simulink model "subsysChanged"  (R2023b)
settings: Solver=VariableStepAuto  StartTime=0.0  StopTime=10.0  RelTol=1e-3
settings Model: Creator=neham  LastModifiedBy=neham

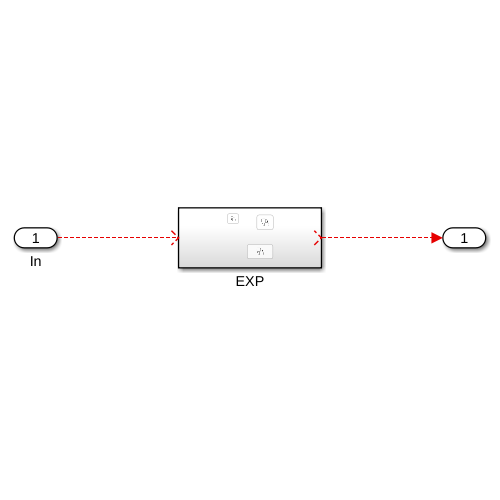
[thumbnail: Simulink's stored preview of the top-level diagram]
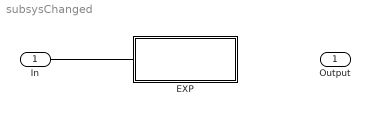
== system subsysChanged ==
  In : Inport
  EXP : Subsystem
  Output : Outport
  wires:
  ? -> Output/1
  In/1 -> ?

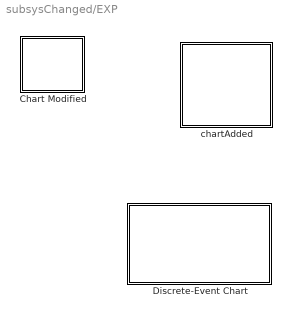
== system subsysChanged/EXP ==
  Chart Modified : Stateflow chart  TreatAsAtomicUnit=on
  Discrete-Event Chart : Stateflow chart  TreatAsAtomicUnit=on
  chartAdded : Stateflow chart  TreatAsAtomicUnit=on

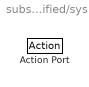
== system subsysChanged/EXP/Chart Modified/sys ==
  Action Port : ActionPort
      settings: CopyFcn=Stateflow.SLINSF.SimulinkMan.removeBlockPreDeleteFcn  PreDeleteFcn=Stateflow.SLINSF.SimulinkMan.unsafePredeleteFcn

== stateflow chart subsysChanged/EXP/chartAdded ==

== stateflow chart subsysChanged/EXP/Chart Modified ==
  state ? [group]
    state ? [function]
      (default) -> (junction 4)
  state sys
  state exp [function]
    (default) -> (junction 13)
  (default) -> sys
  data: sf_internal_action_state_placeholder_data local double size=1 =0
  function adhdh:
    | function adhdh
  function adgdg:
    | function adgdg
    |  
    | 
    | aVarTruthTableCondition_1 = false;
    | 
    | 
    | % sdsdjgs
    | 
    | aVarTruthTableCondition_1 = logical(123);
    | 
    |  % Default
    | 
    | 
    | function aFcnTruthTableAction_1()
    | 
    | % wrsfdkdj
    | 
    | fddg
  function ?:
    | function

== stateflow chart subsysChanged/EXP/Discrete-Event Chart ==
  settings: enableNonTerminalStates=1
